simulink model "TwinRotor_G1_adaptativo"  (Simulink 6.1)
settings: Solver=ode1  SolverMode=SingleTasking  StartTime=0.0  StopTime=45  FixedStep=0.05  RelTol=1e-3
values from neighbouring files (symbols this model uses):
  Kd_tr = 0.01    [def_pid.m]
  Ki_tr = 0.01    [def_pid.m]
  Kp_tr = 0.01    [def_pid.m]
undefined symbols (not defined in the file or in its folder): alpha_theta_1, alpha_theta_2, Gamma_k, Gamma_theta_0, Gamma_theta_1, Gamma_theta_2
libraries: simulink x1, RT x1
settings Model: Creator=Tomás  LastModifiedBy=Zadeh2
settings DataIOCC: SignalLoggingName=sigsOut
settings HardwareCC: TargetEndianess=LittleEndian  TargetHWDeviceType=MATLAB Host  ProdEqTarget=off

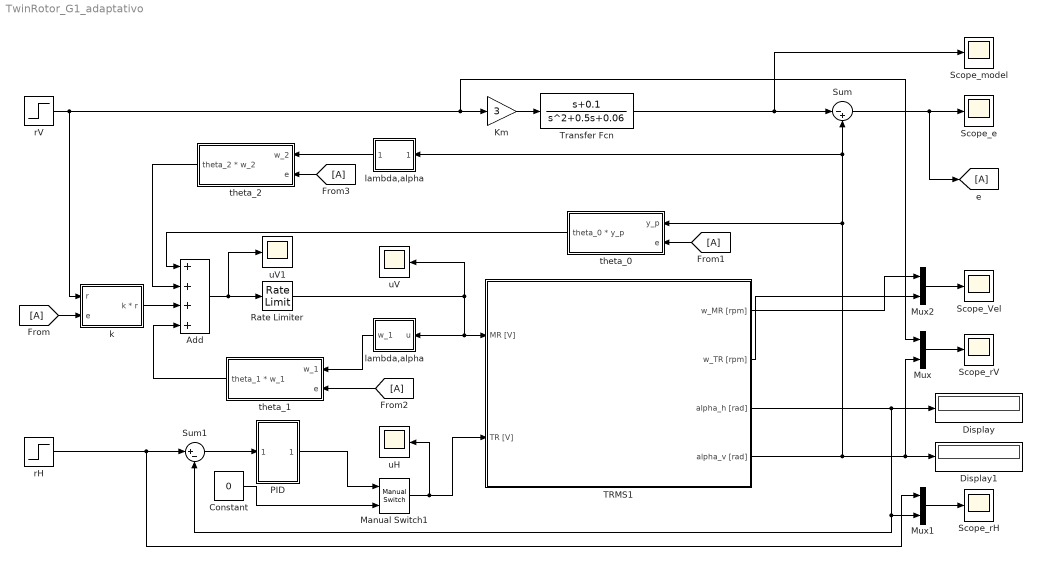
== system TwinRotor_G1_adaptativo ==
  Add : Sum  Inputs=++++  OutDataType=fixdt(1,16,0)  OutScaling=[]
  Constant : Constant  Value=0  OutDataType=fixdt(1,16,0)  OutScaling=[]
  Display : Display
  Display1 : Display
  Km : Gain  Gain=3  ParameterDataType=fixdt(1,16,0)  ParameterScaling=[]  OutDataType=fixdt(1,16,0)  OutScaling=[]
  Manual Switch1 : simulink/Signal Routing/Manual Switch  sw=1  action=0
  Mux : Mux  Inputs=2
  Mux1 : Mux  Inputs=2
  Mux2 : Mux  Inputs=2
  PID : Subsystem
  Rate Limiter : RateLimiter  RisingSlewLimit=2  FallingSlewLimit=-2  SampleTimeMode=inherited
  Scope_Vel : Scope
      settings: YMin=-0.125  YMax=6.125  SaveName=Velocidad  DataFormat=Array  SampleTime=-1
  Scope_e : Scope
      settings: YMin=-38.7875  YMax=-38.73  SaveName=e  DataFormat=Array  SampleTime=-1
  Scope_model : Scope
      settings: YMin=-0.125  YMax=6.125  SaveName=model  DataFormat=Array  SampleTime=-1
  Scope_rH : Scope
      settings: YMin=107.5  YMax=147.5  SaveName=rH  DataFormat=Array  SampleTime=-1
  Scope_rV : Scope
      settings: YMin=-40  YMax=-2.5  SaveName=rV  DataFormat=Array  SampleTime=-1
  Sum : Sum  Inputs=|-+  OutDataType=fixdt(1,16,0)  OutScaling=[]
  Sum1 : Sum  Inputs=|+-  OutDataType=fixdt(1,16,0)  OutScaling=[]
  TRMS1 : Subsystem  mask{Ts=0.05, bias_h=0, bias_v=0, max_mr=20, max_tr=15}
      mask prompts: Ts "Tiempo de Muestreo"; bias_h "bias alpha_h"; bias_v "bias alpha_v"; max_mr "voltaje MR [V]"; max_tr "voltaje TR [V]"
      mask Display:
      | image(imread('Imagenes/Copter.png'))
      | 
      | port_label('output', 1, 'w_MR [rpm]')
      | port_label('output', 2, 'w_TR [rpm]')
      | port_label('output', 3, 'alpha_h [deg]')
      | port_label('output', 4, 'alpha_v [deg]')
      | port_label('input', 1, 'MR [V]')
      | port_label('input', 2, 'TR [V]')
  Transfer Fcn : TransferFcn  Numerator=[1 0.1]  Denominator=[1 0.5 0.06]
  k : Subsystem
  lambda,alpha : Subsystem  Orientation=left
  "lambda,alpha " : Subsystem  Orientation=left
  rH : Step  Time=0  After=140  SampleTime=0
  rV : Step  Time=0  After=-3  SampleTime=0
  theta_0 : Subsystem  Orientation=left
  theta_1 : Subsystem  Orientation=left
  theta_2 : Subsystem  Orientation=left
  uH : Scope
      settings: YMin=-1  YMax=1  SaveName=uH  DataFormat=Array  SampleTime=-1
  uV : Scope
      settings: YMin=0.05  YMax=1.15  SaveName=uV  DataFormat=Array  SampleTime=-1
  uV1 : Scope
      settings: YMin=0  YMax=5000  SaveName=uV1  DataFormat=Array  SampleTime=-1
  wires:
  TRMS1/4(alpha_v [rad]) -> Mux/2, Display1/1, "lambda,alpha "/1(y_p), Sum/2, theta_0/1(y_p)
  TRMS1/3(alpha_h [rad]) -> Display/1, Mux1/2, Sum1/2
  PID/1(Out1) -> Manual Switch1/1
  Constant/1 -> Manual Switch1/2
  Sum1/1 -> PID/1(In1)
  Manual Switch1/1 -> uH/1, TRMS1/2(TR [V])
  rH/1 -> Sum1/1, Mux1/1
  Mux2/1 -> Scope_Vel/1
  Mux/1 -> Scope_rV/1
  Mux1/1 -> Scope_rH/1
  TRMS1/1(w_MR [rpm]) -> Mux2/1
  TRMS1/2(w_TR [rpm]) -> Mux2/2
  Km/1 -> Transfer Fcn/1
  Sum/1 -> [A], Scope_e/1
  Transfer Fcn/1 -> Sum/1, Scope_model/1
  rV/1 -> Mux/1, Km/1, k/1(r)
  theta_0/1(theta_0 * y_p) -> Add/1
  [A] -> theta_0/2(e)
  [A] -> theta_1/2(e)
  [A] -> theta_2/2(e)
  Add/1 -> Rate Limiter/1, uV1/1
  Rate Limiter/1 -> uV/1, lambda,alpha/1(u), TRMS1/1(MR [V])
  theta_1/1(theta_1 * w_1) -> Add/4
  theta_2/1(theta_2 * w_2) -> Add/2
  lambda,alpha/1(w_1) -> theta_1/1(w_1)
  "lambda,alpha "/1(w_2) -> theta_2/1(w_2)
  [A] -> k/2(e)
  k/1(k * r) -> Add/3

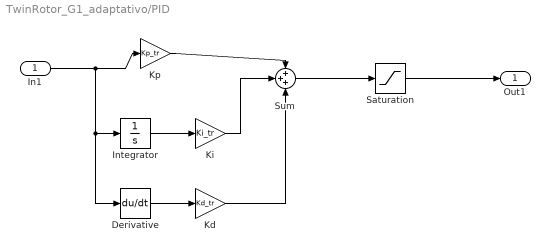
== system TwinRotor_G1_adaptativo/PID ==
  In1 : Inport  Port=1  OutDataType=fixdt(1,16,0)  OutScaling=[]  LatchInput=off
  Derivative : Derivative
  Integrator : Integrator
  Kd : Gain  Gain=Kd_tr  ParameterDataType=fixdt(1,16,0)  ParameterScaling=[]  OutDataType=fixdt(1,16,0)  OutScaling=[]
  Ki : Gain  Gain=Ki_tr  ParameterDataType=fixdt(1,16,0)  ParameterScaling=[]  OutDataType=fixdt(1,16,0)  OutScaling=[]
  Kp : Gain  Gain=Kp_tr  ParameterDataType=fixdt(1,16,0)  ParameterScaling=[]  OutDataType=fixdt(1,16,0)  OutScaling=[]
  Saturation : Saturate  UpperLimit=5  LowerLimit=-5
  Sum : Sum  Inputs=+++  OutDataType=fixdt(1,16,0)  OutScaling=[]
  Out1 : Outport  OutDataType=fixdt(1,16,0)  OutScaling=[]
  wires:
  In1/1 -> Kp/1, Integrator/1, Derivative/1
  Kp/1 -> Sum/1
  Sum/1 -> Saturation/1
  Saturation/1 -> Out1/1
  Integrator/1 -> Ki/1
  Ki/1 -> Sum/2
  Derivative/1 -> Kd/1
  Kd/1 -> Sum/3

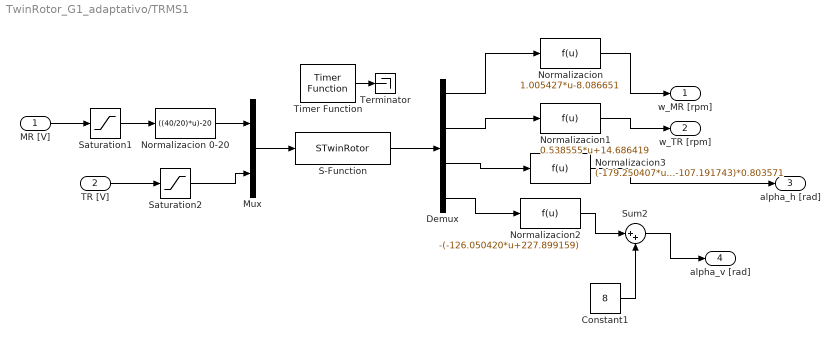
== system TwinRotor_G1_adaptativo/TRMS1 ==
  MR [V] : Inport  Port=1  LatchInput=off
  TR [V] : Inport  Port=2  LatchInput=off
  Constant1 : Constant  Value=8
  Demux : Demux
  Mux : Mux  Inputs=2
  Normalizacion : Fcn  Expr=1.005427*u-8.086651
  Normalizacion 0-20 : Fcn  Expr=((40/20)*u)-20
  Normalizacion1 : Fcn  Expr=0.538555*u+14.686419
  Normalizacion2 : Fcn  Expr=-(-126.050420*u+227.899159)
  Normalizacion3 : Fcn  Expr=(-179.250407*u-107.191743)*0.803571
  S-Function : S-Function  FunctionName=STwinRotor  Parameters=Ts,bias_h,bias_v,max_mr,max_tr
  Saturation1 : Saturate  UpperLimit=20  LowerLimit=0
  Saturation2 : Saturate  UpperLimit=5  LowerLimit=-5
  Sum2 : Sum  Inputs=|++
  Terminator : Terminator
  Timer Function : RT/Timer Function  Priority=777348976  step=50  priority=HIGH  ThPriority=TIME CRITICAL
  w_MR [rpm] : Outport
  w_TR [rpm] : Outport  Port=2
  alpha_h [rad] : Outport  Port=3
  alpha_v [rad] : Outport  Port=4
  wires:
  Constant1/1 -> Sum2/2
  Sum2/1 -> alpha_v [rad]/1
  Normalizacion2/1 -> Sum2/1
  Saturation2/1 -> Mux/2
  Saturation1/1 -> Normalizacion 0-20/1
  Normalizacion3/1 -> alpha_h [rad]/1
  Demux/3 -> Normalizacion3/1
  Demux/4 -> Normalizacion2/1
  Demux/2 -> Normalizacion1/1
  Normalizacion1/1 -> w_TR [rpm]/1
  Demux/1 -> Normalizacion/1
  Normalizacion/1 -> w_MR [rpm]/1
  MR [V]/1 -> Saturation1/1
  Normalizacion 0-20/1 -> Mux/1
  S-Function/1 -> Demux/1
  Mux/1 -> S-Function/1
  TR [V]/1 -> Saturation2/1
  Timer Function/1 -> Terminator/1

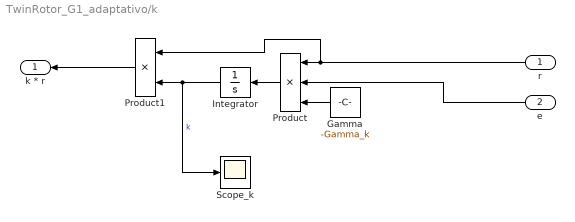
== system TwinRotor_G1_adaptativo/k ==
  r : Inport  Orientation=left  Port=1  OutDataType=fixdt(1,16,0)  OutScaling=[]  LatchInput=off
  e : Inport  Orientation=left  Port=2  OutDataType=fixdt(1,16,0)  OutScaling=[]  LatchInput=off
  Gamma : Constant  Orientation=left  Value=-Gamma_k  OutDataType=fixdt(1,16,0)  OutScaling=[]
  Integrator : Integrator  Orientation=left
  Product : Product  Orientation=left  Inputs=3  OutDataType=fixdt(1,16,0)  OutScaling=[]
  Product1 : Product  Orientation=left  OutDataType=fixdt(1,16,0)  OutScaling=[]
  Scope_k : Scope
      settings: YMin=-10  YMax=10  SaveName=k  DataFormat=Array  SampleTime=-1
  k * r : Outport  Orientation=left  OutDataType=fixdt(1,16,0)  OutScaling=[]
  wires:
  r/1 -> Product1/1, Product/1
  Product1/1 -> k * r/1
  Gamma/1 -> Product/3
  Integrator/1 -> Scope_k/1, Product1/2  "k"
  Product/1 -> Integrator/1
  e/1 -> Product/2

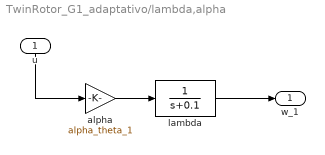
== system TwinRotor_G1_adaptativo/lambda,alpha ==
  u : Inport  Orientation=down  Port=1  OutDataType=fixdt(1,16,0)  OutScaling=[]  LatchInput=off
  alpha : Gain  Gain=alpha_theta_1  ParameterDataType=fixdt(1,16,0)  ParameterScaling=[]  OutDataType=fixdt(1,16,0)  OutScaling=[]
  lambda : TransferFcn  Denominator=[1 0.1]
  w_1 : Outport  OutDataType=fixdt(1,16,0)  OutScaling=[]
  wires:
  alpha/1 -> lambda/1
  u/1 -> alpha/1
  lambda/1 -> w_1/1

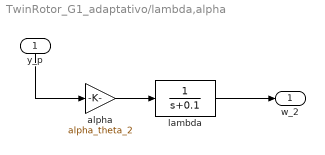
== system TwinRotor_G1_adaptativo/lambda,alpha  ==
  y_p : Inport  Orientation=down  Port=1  OutDataType=fixdt(1,16,0)  OutScaling=[]  LatchInput=off
  alpha : Gain  Gain=alpha_theta_2  ParameterDataType=fixdt(1,16,0)  ParameterScaling=[]  OutDataType=fixdt(1,16,0)  OutScaling=[]
  lambda : TransferFcn  Denominator=[1 0.1]
  w_2 : Outport  OutDataType=fixdt(1,16,0)  OutScaling=[]
  wires:
  alpha/1 -> lambda/1
  y_p/1 -> alpha/1
  lambda/1 -> w_2/1

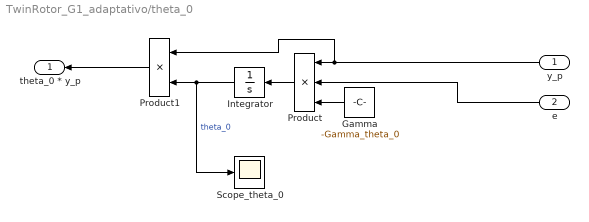
== system TwinRotor_G1_adaptativo/theta_0 ==
  y_p : Inport  Orientation=left  Port=1  OutDataType=fixdt(1,16,0)  OutScaling=[]  LatchInput=off
  e : Inport  Orientation=left  Port=2  OutDataType=fixdt(1,16,0)  OutScaling=[]  LatchInput=off
  Gamma : Constant  Orientation=left  Value=-Gamma_theta_0  OutDataType=fixdt(1,16,0)  OutScaling=[]
  Integrator : Integrator  Orientation=left
  Product : Product  Orientation=left  Inputs=3  OutDataType=fixdt(1,16,0)  OutScaling=[]
  Product1 : Product  Orientation=left  OutDataType=fixdt(1,16,0)  OutScaling=[]
  Scope_theta_0 : Scope
      settings: YMin=-10  YMax=10  SaveName=theta_0  DataFormat=Array  SampleTime=-1
  theta_0 * y_p : Outport  Orientation=left  OutDataType=fixdt(1,16,0)  OutScaling=[]
  wires:
  y_p/1 -> Product1/1, Product/1
  Product1/1 -> theta_0 * y_p/1
  Gamma/1 -> Product/3
  Integrator/1 -> Scope_theta_0/1, Product1/2  "theta_0"
  Product/1 -> Integrator/1
  e/1 -> Product/2

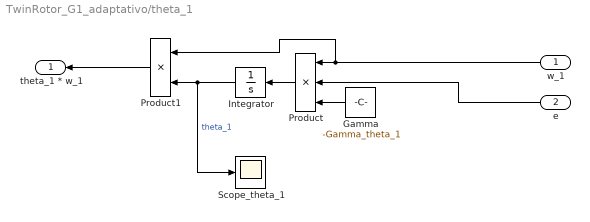
== system TwinRotor_G1_adaptativo/theta_1 ==
  w_1 : Inport  Orientation=left  Port=1  OutDataType=fixdt(1,16,0)  OutScaling=[]  LatchInput=off
  e : Inport  Orientation=left  Port=2  OutDataType=fixdt(1,16,0)  OutScaling=[]  LatchInput=off
  Gamma : Constant  Orientation=left  Value=-Gamma_theta_1  OutDataType=fixdt(1,16,0)  OutScaling=[]
  Integrator : Integrator  Orientation=left
  Product : Product  Orientation=left  Inputs=3  OutDataType=fixdt(1,16,0)  OutScaling=[]
  Product1 : Product  Orientation=left  OutDataType=fixdt(1,16,0)  OutScaling=[]
  Scope_theta_1 : Scope
      settings: YMin=-10  YMax=10  SaveName=theta_1  DataFormat=Array  SampleTime=-1
  theta_1 * w_1 : Outport  Orientation=left  OutDataType=fixdt(1,16,0)  OutScaling=[]
  wires:
  w_1/1 -> Product1/1, Product/1
  Product1/1 -> theta_1 * w_1/1
  Gamma/1 -> Product/3
  Integrator/1 -> Scope_theta_1/1, Product1/2  "theta_1"
  Product/1 -> Integrator/1
  e/1 -> Product/2

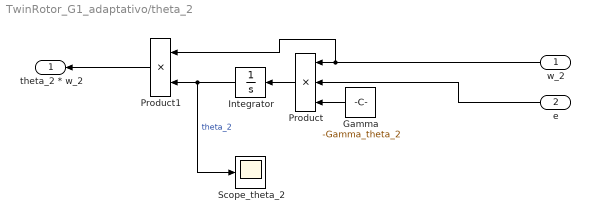
== system TwinRotor_G1_adaptativo/theta_2 ==
  w_2 : Inport  Orientation=left  Port=1  OutDataType=fixdt(1,16,0)  OutScaling=[]  LatchInput=off
  e : Inport  Orientation=left  Port=2  OutDataType=fixdt(1,16,0)  OutScaling=[]  LatchInput=off
  Gamma : Constant  Orientation=left  Value=-Gamma_theta_2  OutDataType=fixdt(1,16,0)  OutScaling=[]
  Integrator : Integrator  Orientation=left
  Product : Product  Orientation=left  Inputs=3  OutDataType=fixdt(1,16,0)  OutScaling=[]
  Product1 : Product  Orientation=left  OutDataType=fixdt(1,16,0)  OutScaling=[]
  Scope_theta_2 : Scope
      settings: YMin=-10  YMax=10  SaveName=theta_2  DataFormat=Array  SampleTime=-1
  theta_2 * w_2 : Outport  Orientation=left  OutDataType=fixdt(1,16,0)  OutScaling=[]
  wires:
  w_2/1 -> Product1/1, Product/1
  Product1/1 -> theta_2 * w_2/1
  Gamma/1 -> Product/3
  Integrator/1 -> Scope_theta_2/1, Product1/2  "theta_2"
  Product/1 -> Integrator/1
  e/1 -> Product/2
